simulink model "sys_dae_tda"  (R2021a)
settings: Solver=daessc  StartTime=0.0  StopTime=20  RelTol=1e-3
settings Model: Creator=Suman  LastModifiedBy=Suman

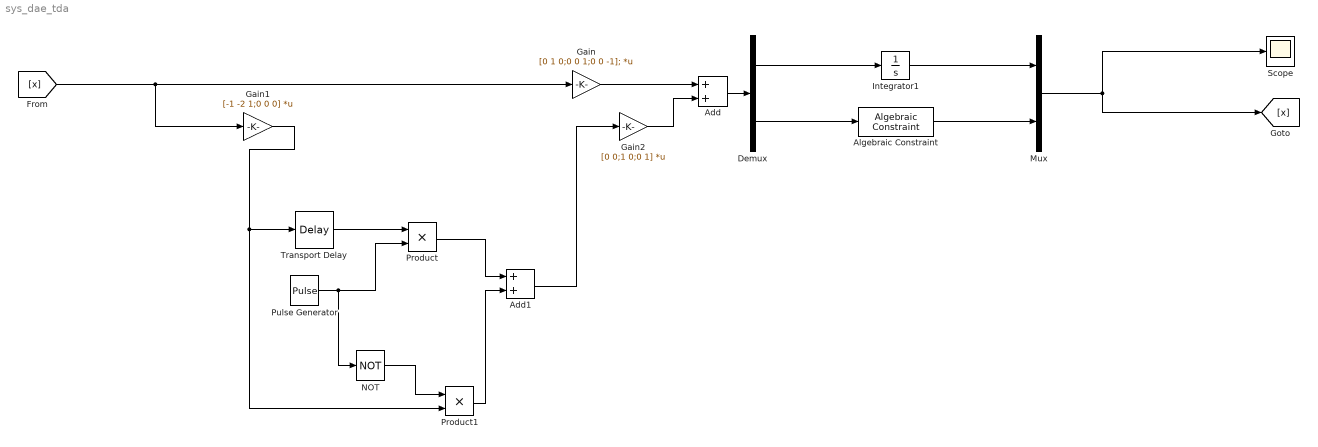
== system sys_dae_tda ==
  Add : Sum
  Add1 : Sum
  Algebraic Constraint : AlgebraicConstraint
  Demux : Demux  Outputs=2
  Gain : Gain  Gain=[0 1 0;0 0 1;0 0 -1];  Multiplication=Matrix(K*u) (u vector)
  Gain1 : Gain  Gain=[-1 -2 1;0 0 0]  Multiplication=Matrix(K*u) (u vector)
  Gain2 : Gain  Gain=[0 0;1 0;0 1]  Multiplication=Matrix(K*u) (u vector)
  Integrator1 : Integrator  InitialCondition=[2;3]
  Mux : Mux  Inputs=2
  NOT : Logic  Operator=NOT  IconShape=distinctive  AllPortsSameDT=off  OutDataTypeStr=boolean
  Product : Product
  Product1 : Product
  Pulse Generator : DiscretePulseGenerator  PulseType=Time based  Period=20  PulseWidth=10  PhaseDelay=3
  Scope : Scope
  Transport Delay : TransportDelay  DelayTime=2
  wires:
  [x] -> Gain1/1, Gain/1
  Gain/1 -> Add/1
  Demux/1 -> Integrator1/1
  Mux/1 -> [x], Scope/1
  Algebraic Constraint/1 -> Mux/2
  Gain2/1 -> Add/2
  Demux/2 -> Algebraic Constraint/1
  Add/1 -> Demux/1
  Integrator1/1 -> Mux/1
  Transport Delay/1 -> Product/1
  Gain1/1 -> Product1/2, Transport Delay/1
  Product/1 -> Add1/1
  Pulse Generator/1 -> NOT/1, Product/2
  NOT/1 -> Product1/1
  Product1/1 -> Add1/2
  Add1/1 -> Gain2/1
